simulink model "model"  (R2016a)
settings: Solver=ode4  StartTime=0.0  StopTime=20  FixedStep=0.001  RelTol=1e-3
settings Model: Creator=Priscilla  LastModifiedBy=Priscilla

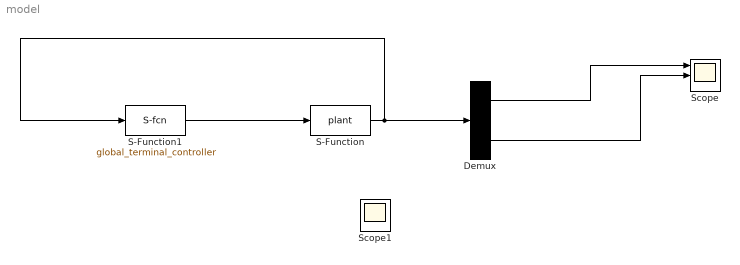
== system model ==
  Demux : Demux  Outputs=2
  S-Function : S-Function  FunctionName=plant  SFunctionDeploymentMode=off  EnableBusSupport=off
  S-Function1 : S-Function  FunctionName=global_terminal_controller  SFunctionDeploymentMode=off  EnableBusSupport=off
  Scope : Scope  NumInputPorts=3
  Scope1 : Scope  NumInputPorts=3
  wires:
  S-Function/1 -> Demux/1, S-Function1/1
  S-Function1/1 -> S-Function/1
  Demux/1 -> Scope/1
  Demux/2 -> Scope/2
